simulink model "A02_L10_1"  (R2021b)
settings: Solver=ode45  StartTime=0.0  StopTime=10  RelTol=1e-3  EnableMultiTasking=on
values from neighbouring files (symbols this model uses):
  k1c = 0.05    [A04_L10_script.m]
  k2c = -0.2    [A04_L10_script.m]
  kwc = 1    [A04_L10_script.m]
settings Model: Creator=User  LastModifiedBy=Adi
settings SolverCC: AlgebraicLoopSolver=TrustRegion
settings DataIOCC: LimitDataPoints=on  SaveFormat=Array  ReturnWorkspaceOutputs=off
settings OptimizationCC: LifeSpan=inf
settings DebuggingCC: SolverPrmCheckMsg=warning  SFUnexpectedBacktrackingDiag=warning  SFNoUnconditionalDefaultTransitionDiag=warning  SFExecutionAtInitializationDiag=none  SFMachineParentedDataDiag=warning  ArithmeticOperatorsInVariantConditions=warning
settings HardwareCC: ProdBitPerPointer=32  ProdBitPerSizeT=32  ProdBitPerPtrDiffT=32  ProdLargestAtomicFloat=None  ProdIntDivRoundTo=Undefined  ProdEndianess=Unspecified  ProdWordSize=32  ProdHWDeviceType=32-bit Generic
settings ModelReferenceCC: PropagateSignalLabelsOutOfModel=off
settings SFSimCC: SimUseLocalCustomCode=off  CustomCodeUndefinedFunction=UseInterfaceOnly
settings RTWCC: RTWUseLocalCustomCode=off
settings CodeAppCC: StateflowObjectComments=on
settings GRTTargetCC: TargetLangStandard=C89/C90 (ANSI)
settings ConfigComp: CovMetricSettings=dw  CovSaveCumulativeToWorkspaceVar=on  CovSaveSingleToWorkspaceVar=on  CovExternalEMLEnable=off  CovSFcnEnable=off

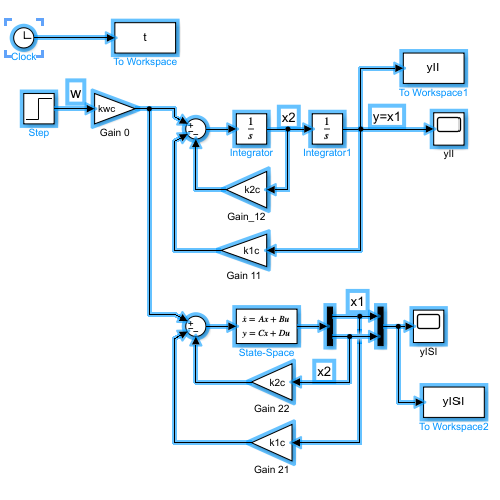
[thumbnail: Simulink's stored preview of the top-level diagram]
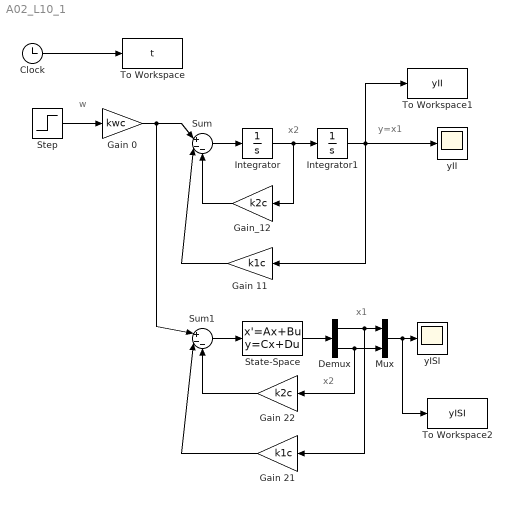
== system A02_L10_1 ==
  note: x1
  note: x2
  note: w
  note: x2
  note: y=x1
  Clock : Clock
  Demux : Demux  Outputs=2
  Gain 0 : Gain  Gain=kwc
  Gain 11 : Gain  Gain=k1c
  Gain 21 : Gain  Gain=k1c
  Gain 22 : Gain  Gain=k2c
  Gain_12 : Gain  Gain=k2c
  Integrator : Integrator
  Integrator1 : Integrator
  Mux : Mux  Inputs=2
  State-Space : StateSpace  A=[0 1;0 0]  B=[0;1]  C=[1 0;0 1]  D=[0;0]  InitialCondition=[0;0]
  Step : Step  Time=0  SampleTime=0
  Sum : Sum  Inputs=|+--
  Sum1 : Sum  Inputs=|+--
  To Workspace : ToWorkspace  VariableName=t  SampleTime=-1
  To Workspace1 : ToWorkspace  VariableName=yII  SampleTime=-1
  To Workspace2 : ToWorkspace  VariableName=yISI  SampleTime=-1
  yII : Scope
  yISI : Scope
  wires:
  Integrator/1 -> Gain_12/1, Integrator1/1
  Sum/1 -> Integrator/1
  Clock/1 -> To Workspace/1
  Step/1 -> Gain 0/1
  Integrator1/1 -> To Workspace1/1, Gain 11/1, yII/1
  Gain_12/1 -> Sum/3
  Gain 11/1 -> Sum/2
  Sum1/1 -> State-Space/1
  Gain 0/1 -> Sum1/1, Sum/1
  Gain 22/1 -> Sum1/3
  Gain 21/1 -> Sum1/2
  State-Space/1 -> Demux/1
  Demux/1 -> Gain 21/1, Mux/1
  Demux/2 -> Gain 22/1, Mux/2
  Mux/1 -> To Workspace2/1, yISI/1
